simulink model "AC"  (R2024b)
settings: Solver=VariableStepAuto  StartTime=0.0  StopTime=inf  RelTol=1e-3
settings Model: Creator=hp  LastModifiedBy=vivan

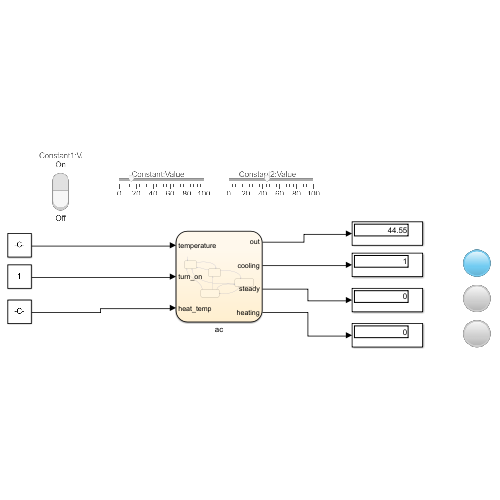
[thumbnail: Simulink's stored preview of the top-level diagram]
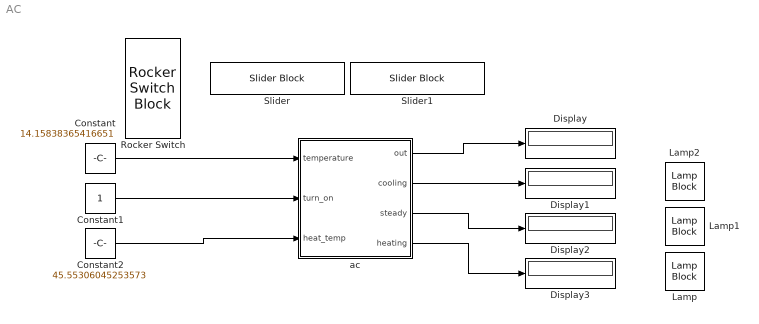
== system AC ==
  Constant : Constant  Value=14.15838365416651
  Constant1 : Constant
  Constant2 : Constant  Value=45.55306045253573
  Display{,1..3} (4 alike) : Display
  Lamp : LampBlock  LabelPosition=Hide
  Lamp1 : LampBlock  LabelPosition=Hide
  Lamp2 : LampBlock  LabelPosition=Hide
  Rocker Switch : RockerSwitchBlock
      settings: Values={{'Off', 'On'}, [0 1]}
  Slider : SliderBlock
  Slider1 : SliderBlock
  ac : Stateflow chart  TreatAsAtomicUnit=on
  wires:
  Constant/1 -> ac/1(temperature)
  Constant1/1 -> ac/2(turn_on)
  ac/1(out) -> Display/1
  Constant2/1 -> ac/3(heat_temp)
  ac/2(cooling) -> Display1/1
  ac/3(steady) -> Display2/1
  ac/4(heating) -> Display3/1

== stateflow chart AC/ac ==
  state on_off
    out=0
  state steady
    out=heat_temp
    steady=1
    cooling=0
    heating=0
  state heat_on
    out=heat_temp+1
    heating=1
    steady=0
    cooling=0
  state cooler_on
    out=heat_temp-1
    cooling=1
    steady=0
    heating=0
  (default) -> on_off : {}
  on_off -> steady : [turn_on==1]
  steady -> on_off [order 2] : [turn_on==0]
  cooler_on -> on_off [order 1] : [turn_on==0]
  heat_on -> on_off [order 1] : [turn_on==0]
  steady -> heat_on [order 1] : [turn_on==1&&...
      | heat_temp<temperature]
  cooler_on -> steady [order 2] : [turn_on==1&&...
      | heat_temp==temperature]
  cooler_on -> heat_on [order 3] : [heat_temp<temperature]
  heat_on -> cooler_on [order 2] : [heat_temp>=temperature]
  data: temperature input; turn_on input; out output; heat_temp input; cooling output; steady output; heating output
